simulink model "Lab_3_model"  (R2024a)
settings: Solver=VariableStepAuto  StartTime=0.0  StopTime=70  MaxStep=0.01  RelTol=1e-4  EnableMultiTasking=on
undefined symbols (not defined in the file or in its folder): comp_gain, den, den_comp, num, num_comp, sensor_constant
libraries: dspsrcs4 x1
settings Model: Creator=Zwivh  LastModifiedBy=Zwivh
settings SolverCC: AlgebraicLoopSolver=TrustRegion
settings DataIOCC: LimitDataPoints=on  SaveOutput=off  SaveTime=off
settings OptimizationCC: ExpressionDepthLimit=2147483647  LifeSpan=1
settings DebuggingCC: UnderspecifiedInitializationDetection=Classic  MergeDetectMultiDrivingBlocksExec=none  FcnCallInpInsideContextMsg=warning  UnconnectedInputMsg=warning  UnconnectedOutputMsg=warning  UnconnectedLineMsg=warning  AllowSymbolicDim=off  StateNameClashWarn=warning  SFUnexpectedBacktrackingDiag=warning  SFNoUnconditionalDefaultTransitionDiag=warning  SFExecutionAtInitializationDiag=none  ArithmeticOperatorsInVariantConditions=warning
settings ModelReferenceCC: EnableRefExpFcnMdlSchedulingChecks=on
settings SFSimCC: SimUseLocalCustomCode=off  CustomCodeUndefinedFunction=UseInterfaceOnly
settings RTWCC: RTWUseLocalCustomCode=off  GPUComputeCapability=3.5
settings CodeAppCC: StateflowObjectComments=on
settings GRTTargetCC: TargetLangStandard=C89/C90 (ANSI)  CombineOutputUpdateFcns=off  GRTInterface=on

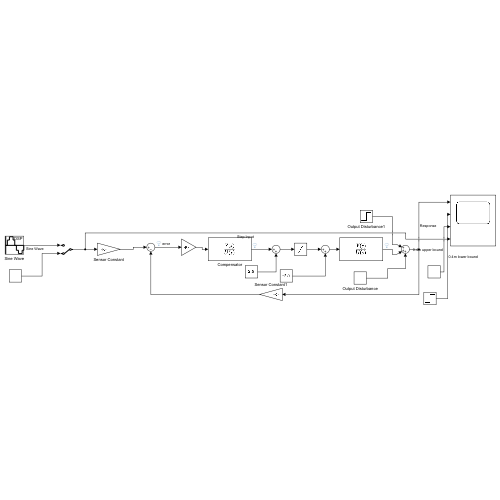
[thumbnail: Simulink's stored preview of the top-level diagram]
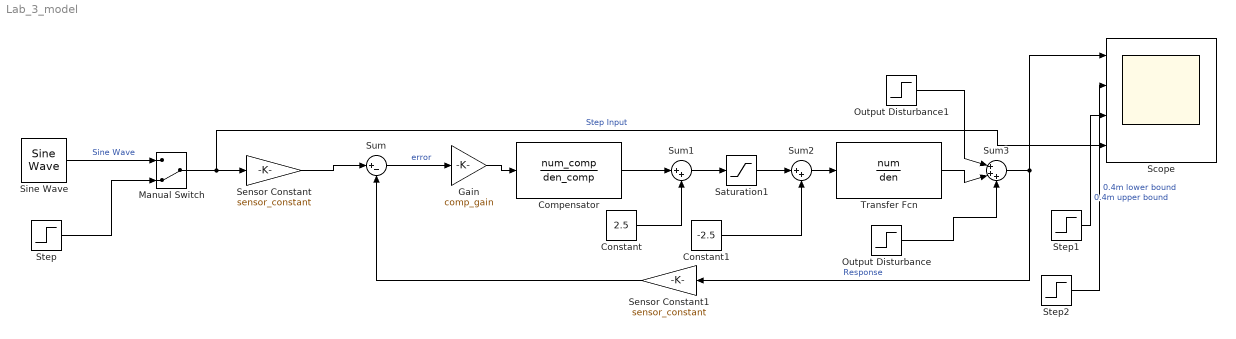
== system Lab_3_model ==
  Compensator : TransferFcn  Numerator=num_comp  Denominator=den_comp
  Constant : Constant  Value=2.5
  Constant1 : Constant  Value=-2.5
  Gain : Gain  Gain=comp_gain
  Manual Switch : ManualSwitch  CurrentSetting=0
  Output Disturbance : Step  Time=7  Before=1  After=0  SampleTime=0
  Output Disturbance1 : Step  Time=13  Before=-1  After=0  SampleTime=0
  Saturation1 : Saturate  UpperLimit=5  LowerLimit=0
  Scope : Scope  NumInputPorts=4
  Sensor Constant : Gain  Gain=sensor_constant
  Sensor Constant1 : Gain  Gain=sensor_constant
  Sine Wave : dspsrcs4/Sine Wave  Amplitude=1  Frequency=0.0159  Phase=0  SampleMode=Discrete  OutComplex=Real  CompMethod=Trigonometric fcn  TableSize=Speed  SampleTime=1/1000  SamplesPerFrame=1  ResetState=Restart at time zero  OutputFrames=off  dataType=double  wordLen=16  udDataType=sfix(16)  fracBitsMode=Best precision  numFracBits=15  OutDataTypeStr=double  LastOutDataTypeStr=double
  Step : Step  After=5  SampleTime=0
  Step1 : Step  After=5.4  SampleTime=0
  Step2 : Step  After=4.6  SampleTime=0
  Sum : Sum  Inputs=|+-
  Sum1 : Sum  Inputs=|++
  Sum2 : Sum  Inputs=|++
  Sum3 : Sum  Inputs=|+++
  Transfer Fcn : TransferFcn  Numerator=num  Denominator=den
  wires:
  Sum/1 -> Gain/1  "error"
  Sensor Constant1/1 -> Sum/2
  Compensator/1 -> Sum1/1
  Constant/1 -> Sum1/2
  Constant1/1 -> Sum2/2
  Sensor Constant/1 -> Sum/1
  Saturation1/1 -> Sum2/1
  Sum2/1 -> Transfer Fcn/1
  Sum1/1 -> Saturation1/1
  Gain/1 -> Compensator/1
  Transfer Fcn/1 -> Sum3/2
  Sum3/1 -> Sensor Constant1/1, Scope/1  "Response"
  Manual Switch/1 -> Scope/4, Sensor Constant/1  "Step Input"
  Sine Wave/1 -> Manual Switch/1  "Sine Wave"
  Step/1 -> Manual Switch/2
  Output Disturbance/1 -> Sum3/3
  Output Disturbance1/1 -> Sum3/1
  Step1/1 -> Scope/3  "0.4m upper bound"
  Step2/1 -> Scope/2  "0.4m lower bound"
